simulink model "matlab_function_complex_test"  (Simulink 8.4)
settings: Solver=ode45  StartTime=0.0  StopTime=10.0  RelTol=1e-3
settings Model: Creator=arnaud  LastModifiedBy=arnaud
settings DataIOCC: SaveFormat=Structure  SignalLoggingSaveFormat=Dataset
settings OptimizationCC: ExpressionDepthLimit=128
settings DebuggingCC: UnderspecifiedInitializationDetection=Simplified  MergeDetectMultiDrivingBlocksExec=error  FcnCallInpInsideContextMsg=EnableAllAsError  StateNameClashWarn=none
settings GRTTargetCC: CombineOutputUpdateFcns=on  GRTInterface=off

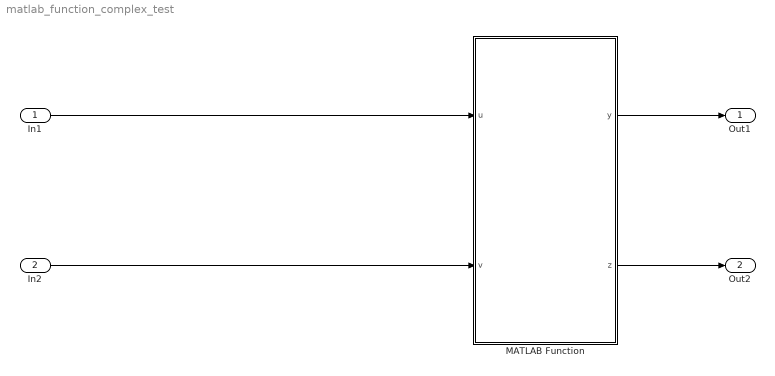
== system matlab_function_complex_test ==
  In1 : Inport  OutDataTypeStr=double  PortDimensions=1  BusOutputAsStruct=on
      settings: SignalType=complex
  In2 : Inport  Port=2  OutDataTypeStr=double  PortDimensions=1
      settings: SignalType=complex
  MATLAB Function : MATLAB Function  TreatAsAtomicUnit=on
  Out1 : Outport
  Out2 : Outport  Port=2
  wires:
  In1/1 -> MATLAB Function/1(u)
  In2/1 -> MATLAB Function/2(v)
  MATLAB Function/1(y) -> Out1/1
  MATLAB Function/2(z) -> Out2/1

== matlab function MATLAB Function ==
  data: u input double; y output double; v input double; z output double
function [y, z] = do_stuff(u, v)
%#codegen

y = u;
z = v;
